simulink model "DataGeneration_ExampleIII"  (Simulink 2.20)
settings: Solver=ode5  StartTime=0.0  StopTime=85500  FixedStep=0.0025  RelTol=1e-3  AbsTol=1e-6
libraries: DABLib x1
settings Model: ConsistencyChecking=off  RTWPlaceOutputsASAP=off

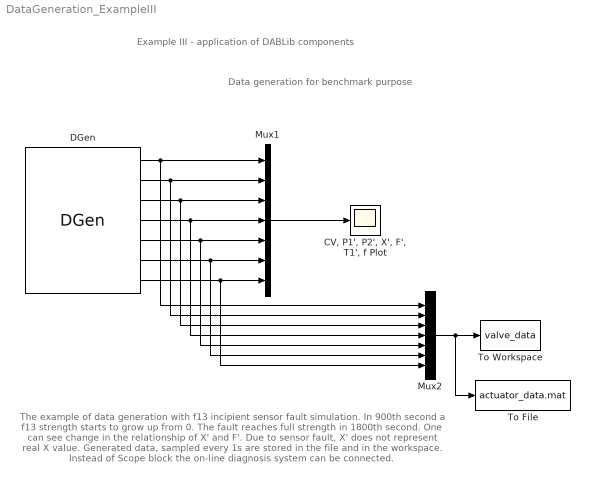
== system DataGeneration_ExampleIII ==
  note: Data generation for benchmark purpose
  note: Example III - application of DABLib components
  note: The example of data generation with f13 incipient sensor fault simulation.
      | In 900th second a f13 strength starts to grow up from 0.
      | The fault reaches full strength in 1800th second.
      | One can see change in the relationship of X' and F'.
      | Due to sensor fault, X' does not represent real X value.
      | Generated data, sampled every 1s are stored in the file and in the workspace.
      | Instead of Scope block the on-line diagnosis system can be connected.
  "CV, P1', P2', X', F', T1', f Plot" : Scope
      settings: TickLabels=on  TimeRange=2100  YMin=0  YMax=1  SaveToWorkspace=off  SaveName=ScopeData  MaxRows=3600  SampleInput=on  SampleTime=1
  DGen : DABLib/DGen  FSel=f13 - Rod displacement sensor fault  FType=Incipient
  Mux1 : Mux  Inputs=7
  Mux2 : Mux  Inputs=7
  To File : ToFile  Filename=actuator_data.mat  MatrixName=actuator_data  SampleTime=1
  To Workspace : ToWorkspace  VariableName=valve_data  SampleTime=1
  wires:
  Mux1/1 -> "CV, P1', P2', X', F', T1', f Plot"/1
  DGen/7 -> Mux2/7, Mux1/7
  DGen/6 -> Mux2/6, Mux1/6
  DGen/5 -> Mux1/5, Mux2/5
  DGen/3 -> Mux2/3, Mux1/3
  DGen/2 -> Mux2/2, Mux1/2
  DGen/1 -> Mux1/1, Mux2/1
  DGen/4 -> Mux1/4, Mux2/4
  Mux2/1 -> To Workspace/1, To File/1
